simulink model "Rack and Pinion Model"  (R2022b)
settings: Solver=VariableStepAuto  StartTime=0.0  StopTime=20  RelTol=1e-3
values from neighbouring files (symbols this model uses):
  b1 = 10    [SimWorkSpace.mat]
  b2 = 10    [SimWorkSpace.mat]
  J = 10    [SimWorkSpace.mat]
  k1 = 10    [SimWorkSpace.mat]
  k2 = 10    [SimWorkSpace.mat]
  m = 1    [SimWorkSpace.mat]
  R = 0.5    [SimWorkSpace.mat]
settings Model: Creator=frz  LastModifiedBy=frz

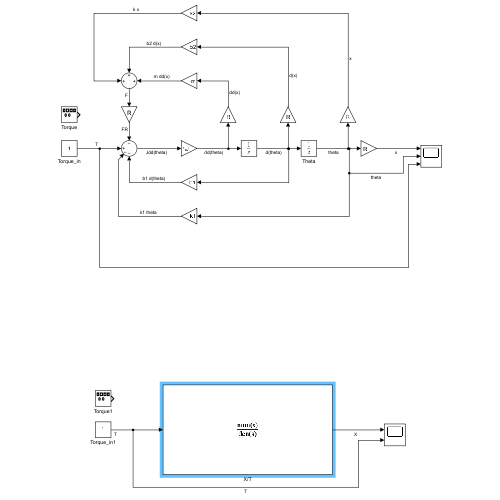
[thumbnail: Simulink's stored preview of the top-level diagram]
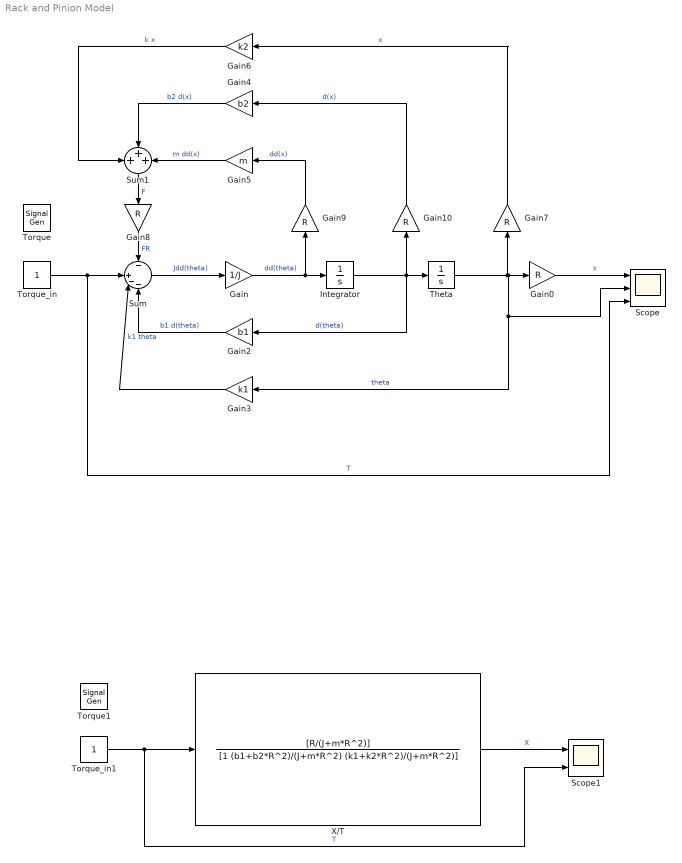
== system Rack and Pinion Model ==
  Gain : Gain  Gain=1/J
  Gain{0,7..10} (5 alike) : Gain  Gain=R
  Gain2 : Gain  Gain=b1
  Gain3 : Gain  Gain=k1
  Gain4 : Gain  Gain=b2
  Gain5 : Gain  Gain=m
  Gain6 : Gain  Gain=k2
  Integrator : Integrator
  Scope : Scope  NumInputPorts=3
  Scope1 : Scope  NumInputPorts=2
  Sum : Sum  Inputs=-|+--
  Sum1 : Sum  Inputs=+++
  Theta : Integrator
  Torque : SignalGenerator  Units=rad/sec
  Torque1 : SignalGenerator  Units=rad/sec
  Torque_in : Constant
  Torque_in1 : Constant
  X/T : TransferFcn  Numerator=[R/(J+m*R^2)]  Denominator=[1 (b1+b2*R^2)/(J+m*R^2) (k1+k2*R^2)/(J+m*R^2)]
  wires:
  Sum/1 -> Gain/1  "Jdd(theta)"
  Sum1/1 -> Gain8/1  "F"
  Gain/1 -> Gain9/1, Integrator/1  "dd(theta)"
  Integrator/1 -> Gain2/1, Theta/1, Gain10/1  "d(theta)"
  Theta/1 -> Gain3/1, Scope/2, Gain0/1, Gain7/1  "theta"
  Gain0/1 -> Scope/1  "x"
  Gain2/1 -> Sum/4  "b1 d(theta)"
  Gain3/1 -> Sum/3  "k1 theta"
  Gain5/1 -> Sum1/3  "m dd(x)"
  Gain4/1 -> Sum1/2  "b2 d(x)"
  Gain6/1 -> Sum1/1  "k x"
  Gain8/1 -> Sum/1  "FR"
  Gain9/1 -> Gain5/1  "dd(x)"
  Gain10/1 -> Gain4/1  "d(x)"
  Gain7/1 -> Gain6/1  "x"
  Torque_in/1 -> Scope/3, Sum/2  "T"
  X/T/1 -> Scope1/1  "X"
  Torque_in1/1 -> Scope1/2, X/T/1  "T"
